simulink model "BitwiseAND_int8"  (R2017b)
settings: Solver=ode3  StartTime=0.0  StopTime=10.0  FixedStep=0.200000  RelTol=1e-3
libraries: simulink x3
settings Model: Creator=hbourbou  LastModifiedBy=hbourbou
settings OptimizationCC: LifeSpan=inf
settings DebuggingCC: SFExecutionAtInitializationDiag=none
settings HardwareCC: ProdBitPerSizeT=32  ProdBitPerPtrDiffT=32  ProdWordSize=32  ProdHWDeviceType=Specified
settings CodeAppCC: StateflowObjectComments=on

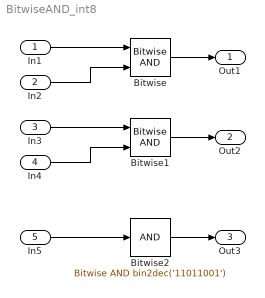
== system BitwiseAND_int8 ==
  In1 : Inport  OutDataTypeStr=int8
  In2 : Inport  Port=2  OutDataTypeStr=int8
  In3 : Inport  Port=3  OutDataTypeStr=int8
  In4 : Inport  Port=4  OutDataTypeStr=int8  PortDimensions=3
  In5 : Inport  Port=5  OutDataTypeStr=int8  PortDimensions=3
  Bitwise : simulink/Logic and Bit Operations/Bitwise Operator  logicop=AND  UseBitMask=off  NumInputPorts=2  BitMask=bin2dec('11011001')  BitMaskRealWorld=Stored Integer
  Bitwise1 : simulink/Logic and Bit Operations/Bitwise Operator  logicop=AND  UseBitMask=off  NumInputPorts=2  BitMask=bin2dec('11011001')  BitMaskRealWorld=Stored Integer
  Bitwise2 : simulink/Logic and Bit Operations/Bitwise Operator  logicop=AND  UseBitMask=on  BitMask=bin2dec('11011001')  BitMaskRealWorld=Stored Integer
  Out1 : Outport
  Out2 : Outport  Port=2
  Out3 : Outport  Port=3
  wires:
  In1/1 -> Bitwise/1
  In2/1 -> Bitwise/2
  Bitwise/1 -> Out1/1
  Bitwise1/1 -> Out2/1
  In3/1 -> Bitwise1/1
  In4/1 -> Bitwise1/2
  In5/1 -> Bitwise2/1
  Bitwise2/1 -> Out3/1
